simulink model "tipy_double_mujoco"  (R2026a)
settings: Solver=FixedStepDiscrete  StopTime=10  FixedStep=0.0050000000000000001
libraries: mjLib x1

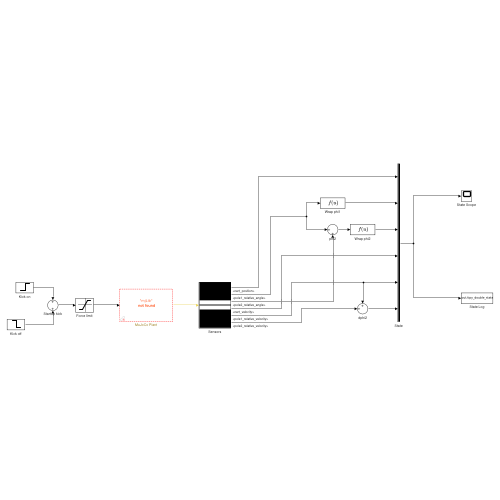
[thumbnail: Simulink's stored preview of the top-level diagram]
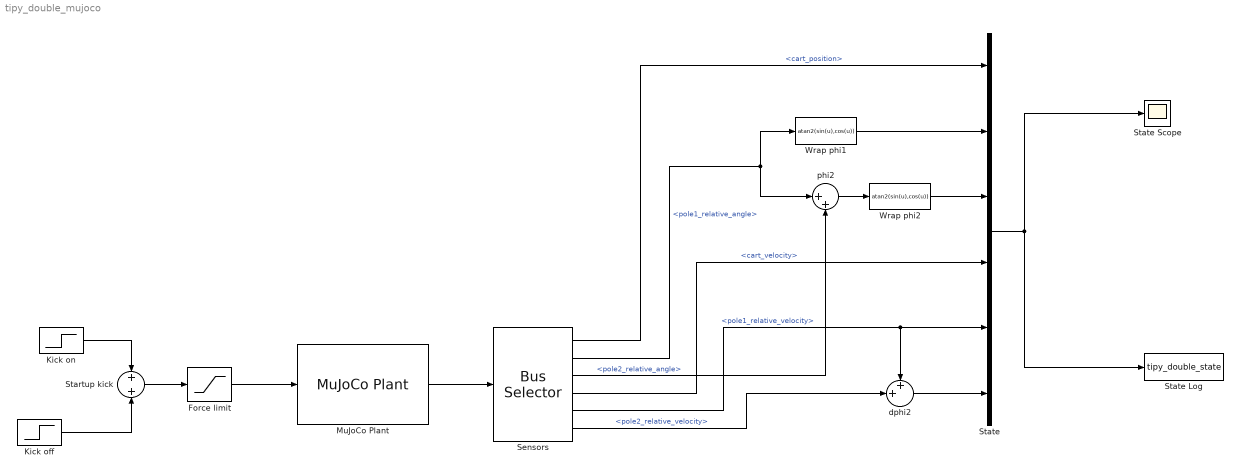
== system tipy_double_mujoco ==
  Force limit : Saturate  UpperLimit=20  LowerLimit=-20
  Kick off : Step  Time=0.050000000000000003  FinalValue=-1  SampleTime=0
  Kick on : Step  Time=0  SampleTime=0
  MuJoCo Plant : mjLib/MuJoCo Plant  controlBus=[]  sensorBus=mj_bus_sensor_7979902499018342666  controlLength=[]  sensorLength=[]  rgbLength=[]  depthLength=[]  sampleTime=0.005  xmlFileRel=/home/matlab/work/Tipy/src/double/model.xml  xmlFile=/home/matlab/work/Tipy/src/double/model.xml  renderingType=Global  vsync=off  visualFPS=60  zoomLevel=1  znear=0.042401  zfar=212.0061  cameraSampleTime=0.020  rgbOutOption=on  depthOutOption=off  controlInterfaceType=Vector
      settings: SourceProductName=MuJoCo Simulator
  Sensors : BusSelector  OutputSignals=cart_position,pole1_relative_angle,pole2_relative_angle,cart_velocity,pole1_relative_velocity,pole2_relative_velocity
  Startup kick : Sum
  State : Mux  Inputs=6
  State Log : ToWorkspace  VariableName=tipy_double_state  SampleTime=-1
  State Scope : Scope
  Wrap phi1 : Fcn  Expr=atan2(sin(u),cos(u))
  Wrap phi2 : Fcn  Expr=atan2(sin(u),cos(u))
  dphi2 : Sum  Inputs=++|
  phi2 : Sum  Inputs=|++
  wires:
  Kick on/1 -> Startup kick/1
  Kick off/1 -> Startup kick/2
  Startup kick/1 -> Force limit/1
  Force limit/1 -> MuJoCo Plant/1
  MuJoCo Plant/1 -> Sensors/1
  Sensors/2 -> Wrap phi1/1, phi2/1  "<pole1_relative_angle>"
  Sensors/3 -> phi2/2  "<pole2_relative_angle>"
  Sensors/5 -> dphi2/1, State/5  "<pole1_relative_velocity>"
  Sensors/6 -> dphi2/2  "<pole2_relative_velocity>"
  phi2/1 -> Wrap phi2/1
  Sensors/1 -> State/1  "<cart_position>"
  Wrap phi1/1 -> State/2
  Wrap phi2/1 -> State/3
  Sensors/4 -> State/4  "<cart_velocity>"
  dphi2/1 -> State/6
  State/1 -> State Log/1, State Scope/1
